simulink model "untitled2"  (R2018b)
settings: Solver=VariableStepAuto  StartTime=0.0  StopTime=5  RelTol=1e-3
libraries: commutil2 x2, dspquant2 x2, dsparch4 x1, dspsigops x1
settings Model: Creator=nhat  LastModifiedBy=nhat

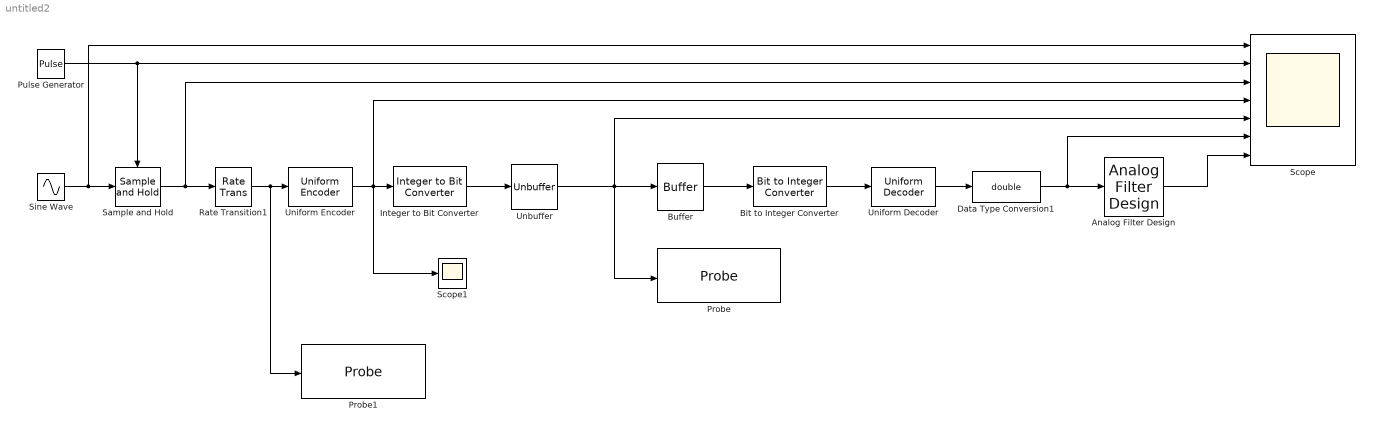
== system untitled2 ==
  Analog Filter Design : dsparch4/Analog Filter Design  method=Butterworth  filttype=Lowpass  N=8  Wlo=3100*2*pi  Whi=80  Rp=2  Rs=40
  Bit to Integer Converter : commutil2/Bit to Integer Converter  nbits=8  bitOrder=MSB first  signedOutputValues=Unsigned  outDtype=Inherit via internal rule  outDtypeSigned=Inherit via internal rule
  Buffer : Buffer  N=8  OutputFrames=off
  Data Type Conversion1 : DataTypeConversion  OutDataTypeStr=double
  Integer to Bit Converter : commutil2/Integer to Bit Converter  nbits=8  signedInputValues=Unsigned  bitOrder=MSB first  outDtype=Inherit via internal rule
  Probe : Probe  ProbeSignalDimensions=on  ProbeWidthDataType=Same as input  ProbeSampleTimeDataType=Same as input  ProbeComplexityDataType=Same as input  ProbeDimensionsDataType=Same as input
  Probe1 : Probe  ProbeSignalDimensions=on  ProbeWidthDataType=Same as input  ProbeSampleTimeDataType=Same as input  ProbeComplexityDataType=Same as input  ProbeDimensionsDataType=Same as input
  Pulse Generator : DiscretePulseGenerator  PulseType=Time based  Period=1/8000  PulseWidth=50
  Rate Transition1 : RateTransition  OutPortSampleTime=1/8000
  Sample and Hold : dspsigops/Sample and Hold  trig=Rising edge  initCond=0  latchinput=off
  Scope : Scope  NumInputPorts=7
  Scope1 : Scope
  Sine Wave : Sin  Frequency=3000*2*pi  SampleTime=1/64000
  Unbuffer : Unbuffer
  Uniform Decoder : dspquant2/Uniform Decoder  peak=1  bits=8  overflowMode=Saturate  otype=Double
      settings: SourceProductName=DSP System Toolbox  SourceProductBaseCode=DS
  Uniform Encoder : dspquant2/Uniform Encoder  peak=1  bits=8  otype=Unsigned integer
      settings: SourceProductName=DSP System Toolbox
  wires:
  Sine Wave/1 -> Scope/1, Sample and Hold/1
  Sample and Hold/1 -> Scope/3, Rate Transition1/1
  Rate Transition1/1 -> Probe1/1, Uniform Encoder/1
  Integer to Bit Converter/1 -> Unbuffer/1
  Pulse Generator/1 -> Sample and Hold/Trigger, Scope/2
  Uniform Encoder/1 -> Scope1/1, Scope/4, Integer to Bit Converter/1
  Unbuffer/1 -> Scope/5, Buffer/1, Probe/1
  Buffer/1 -> Bit to Integer Converter/1
  Bit to Integer Converter/1 -> Uniform Decoder/1
  Uniform Decoder/1 -> Data Type Conversion1/1
  Data Type Conversion1/1 -> Scope/6, Analog Filter Design/1
  Analog Filter Design/1 -> Scope/7
